simulink model "electrical_model_validation_2015"  (R2015a)
settings: Solver=ode4  StartTime=0.0  StopTime=inf  FixedStep=0.001  RelTol=1e-3
libraries: PoliArd x7
settings Model: CovHtmlReporting=off  ExtModeTrigDuration=2  Creator=User  LastModifiedBy=User
settings OptimizationCC: OptimizeModelRefInitCode=on  LifeSpan=1
settings DebuggingCC: UnderspecifiedInitializationDetection=Classic  MergeDetectMultiDrivingBlocksExec=none
settings HardwareCC: ProdLargestAtomicInteger=Long  ProdLargestAtomicFloat=Double  ProdEndianess=LittleEndian  ProdHWDeviceType=ARM Compatible->ARM Cortex
settings RTWCC: SystemTargetFile=realtime.tlc  GenerateMakefile=off  TemplateMakefile=realtime.tmf  Description=Run on Target Hardware  RTWVerbose=off
settings ERTTargetCC: CombineOutputUpdateFcns=off  ExtModeTransport=3  ExtModeMexFile=ext_serial_win32_comm_rtt  ExtModeMexArgs=0 1 9600  InlinedParameterPlacement=Hierarchical  ERTSrcFileBannerTemplate=realtime_code_template.cgt  ERTHdrFileBannerTemplate=realtime_code_template.cgt  ERTDataSrcFileTemplate=realtime_code_template.cgt  ERTDataHdrFileTemplate=realtime_code_template.cgt  ERTCustomFileTemplate=realtime_file_process.tlc

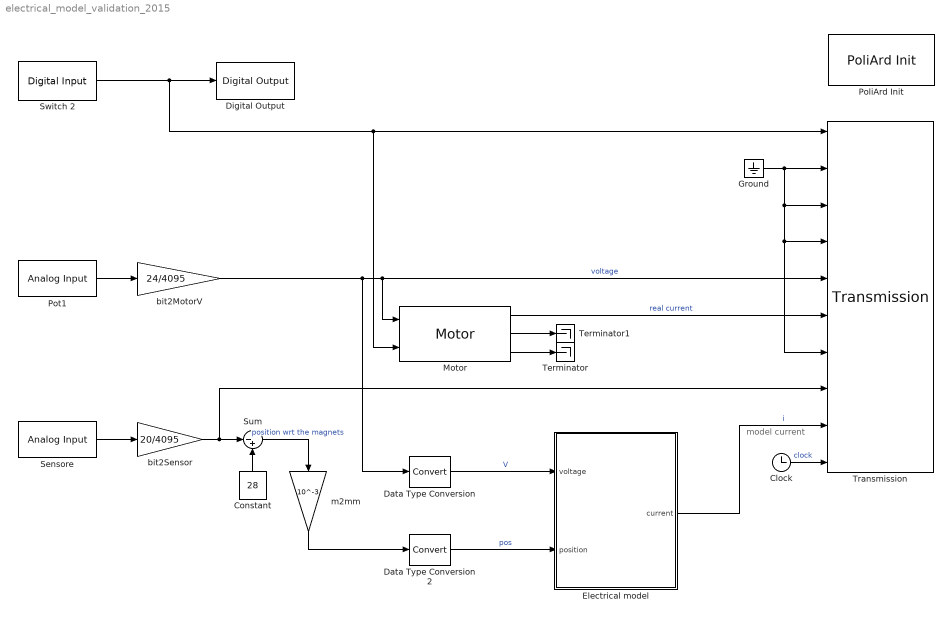
== system electrical_model_validation_2015 ==
  note: model current
  Clock : Clock
  Constant : Constant  Value=28
  Data Type Conversion : DataTypeConversion
  Data Type Conversion2 : DataTypeConversion
  Digital Output : PoliArd/Digital Output  DO_pin=1
  Electrical model : Subsystem
      mask Display: disp('Electrical\nmodel')
  Ground : Ground
  Motor : PoliArd/Motor  MotorID=2  DC_bus_mask=24  dt_mot=-1
  PoliArd Init : PoliArd/PoliArd Init
  Pot1 : PoliArd/Analog Input  AIpin_mask=8  AIsample=-1
  Sensore : PoliArd/Analog Input  AIpin_mask=2  AIsample=-1
  Sum : Sum  Inputs=|-+
  Switch 2 : PoliArd/Digital Input  DI_pin=2  DIsample=-1
  Terminator : Terminator
  Terminator1 : Terminator
  Transmission : PoliArd/Transmission  sample_freq=100  sig_to_send=6
  bit2MotorV : Gain  Gain=24/4095
  bit2Sensor : Gain  Gain=20/4095
  m2mm : Gain  Gain=10^-3
  wires:
  Switch 2/1 -> Motor/2, Transmission/1, Digital Output/1
  Pot1/1 -> bit2MotorV/1
  bit2MotorV/1 -> Data Type Conversion/1, Motor/1, Transmission/5  "voltage"
  Sensore/1 -> bit2Sensor/1
  Ground/1 -> Transmission/7, Transmission/4, Transmission/3, Transmission/2
  Motor/1 -> Transmission/6  "real current"
  Data Type Conversion/1 -> Electrical model/1(voltage)  "V"
  Data Type Conversion2/1 -> Electrical model/2(position)  "pos"
  Electrical model/1(current) -> Transmission/9  "i"
  bit2Sensor/1 -> Transmission/8, Sum/1
  Constant/1 -> Sum/2
  Sum/1 -> m2mm/1  "position wrt the magnets"
  m2mm/1 -> Data Type Conversion2/1
  Clock/1 -> Transmission/10  "clock"
  Motor/3 -> Terminator/1
  Motor/2 -> Terminator1/1

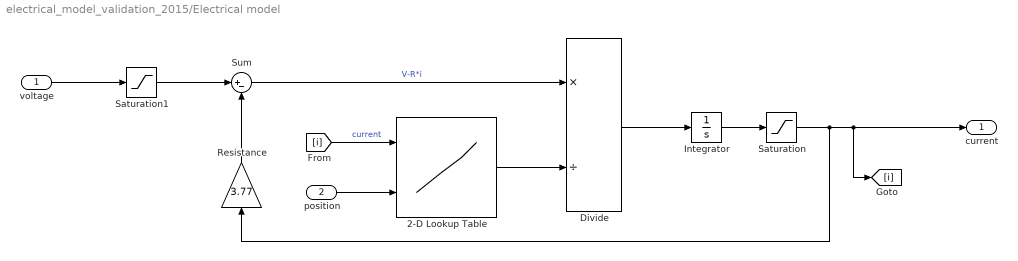
== system electrical_model_validation_2015/Electrical model ==
  voltage : Inport
  position : Inport  Port=2
  2-D Lookup Table : Lookup_n-D  BreakpointsForDimension1="[0.571609272941941\t0.887378665517721\t1.20335132735163\t1.45876147710325\t1.73983455991042\t2.00390586430628\t2.24859052314101\t2.53711534582031\t2.81056000291084\t3.07646645256203\t3.35127777604811\t3.64723023514144\t3.85000000000000]"  BreakpointsForDimension2="[0.00850000000000000\t0.00970000000000000\t0.0105000000000000\t0.0113000000000000\t0.0125000000000000\t0.0135000000000000\t0.0145000000000000\t0.0153000000000000\t0.0165000000000000\t0.0176000000000000\t0.0183000000000000\t0.0198000000000000\t0.0216000000000000\t0.0227000000000000\t0.0236000000000000\t0.0250000000000000]"  Table=|  InternalRulePriority=Speed  RndMeth=Simplest  InputSameDT=on
      | [0.124059778904572	0.115240241777071	0.113604140674407	0.0969706688265998	0.0977224474024037	0.0921484095955819	0.100328887428518	0.0835138746623809	0.0846632562500726	0.101320516519449	0.0850868072661021	0.0849911313704199	0.0770233226672402	0.0728199039666389	0.0857349673426359	0.0658782797079401;
      | 0.149045221919738	0.116659637086155	0.0895561667908866	0.107893626307192	0.125389770928968	0.115549357372873	0.107628431471634	0.0767478700757045	0.113734620814557	0.0487030540411753	0.0854166029154558	0.0852375799265393	0.114494610905458	0.0825536179015005	0.0749113685323473	0.0864552033453527;
      | 0.221473301610230	0.138359268104424	0.127598655408847	0.107655509943492	0.141088050151794	0.102255183896598	0.103076473457404	0.0872435174437226	0.0836166062440565	0.0888634655755324	0.0932839743614151	0.0915177204990435	0.132016146787556	0.0970366780879440	0.0904130771398634	0.108966956576679;
      | 0.223991273176650	0.131524925501924	0.123595637192268	0.117399436946038	0.117485034279105	0.109350617361035	0.103754507171467	0.0861589388580345	0.0857214364348041	0.0917816549943483	0.0890067546609038	0.0816722200620728	0.0814610836052316	0.0767116899255463	0.101900659316609	0.0822633503211632;
      | 0.121687886024072	0.142564456752788	0.125484097705187	0.149105978672514	0.0988303311903818	0.106857219213140	0.0894649045582189	0.0941267712338361	0.142565468524165	0.0818497060473378	0.118301103228728	0.108957534804165	0.106456207125703	0.0760919077107217	0.100144658956964	0.0822619257219681;
      | 0.136138515173081	0.131275746991678	0.174923869014491	0.116373234031288	0.134897498149436	0.147488603603662	0.117217593568497	0.121092621011354	0.0949684484680815	0.120650625212044	0.105528056130615	0.0709218655223650	0.106865162540236	0.112621349170388	0.102672846353554	0.0998828162723997;
      | 0.102540529062246	0.129063716207047	0.128781249629223	0.166531606601018	0.160188607891842	0.143350181522525	0.115424867410468	0.0924580701157953	0.0820347096702044	0.143659809333330	0.0960185227869846	0.0879236610127591	0.119698929732948	0.104624971346943	0.110768236008707	0.103967680724277;
      | 0.0502869330876773	0.0703360930295036	0.121482000910445	0.0868865611541192	0.0998730250371566	0.116253725751726	0.167400667443646	0.161303839871314	0.0985175204299240	0.108488089108738	0.109759635054218	0.0872452567890512	0.125353645131964	0.0875259849372003	0.0849935304722978	0.121626189232489;
      | 0.0210706133138075	0.0515351091202676	0.0426200646343306	0.0565782276211947	0.0745690977819913	0.112020657359165	0.119725047783217	0.0764647313692596	0.142348650861394	0.0639349050075603	0.0904353025903782	0.0861112460202275	0.104664668411399	0.0920235686672933	0.100744620630661	0.106708466661268;
      | 0.0270141671779473	0.0514415556627170	0.0517146134495731	0.0520472356443474	0.0605274494443696	0.0377197714304948	0.0779920314933253	0.0546966093282379	0.106915061624985	0.0869951773796697	0.0883601743545483	0.0742534146214650	0.0717300175437439	0.0897862727514690	0.0997181913290360	0.104066264542440;
      | 0.0233295954754315	0.0449998739143449	0.0266561560962006	0.0155280944859940	0.0317770292575240	0.0319196439820041	0.0527561841503626	0.0297736212828209	0.0370581914149013	0.0386385191066780	0.0587271929401315	0.0453068226188899	0.0773245158334478	0.0738659266965119	0.0647672762562245	0.0535420982543080;
      | 0.0413476484233245	0.0276536768519413	0.0409781731998001	0.0196987497152002	0.0318266325664729	0.0299424263688483	0.0360092728529738	0.0227687678372619	0.0349869001320810	0.0443660538458634	0.0517921958134473	0.0205963949400280	0.0348039807615572	0.0511089243845314	0.0453265105118442	0.0715060082844046;
      | 0.0130190041072452	0.0146415091158683	0.0254138121892464	0.0412159054731432	0.0223960404799849	0.0227241118668500	0.0456462201437789	0.0149368008701184	0.0420919416421131	0.0187588708287234	0.0329663489886674	0.0687911911872538	0.0275417699258336	0.0252373999239683	0.0212106687462740	0.0791031180455345]
  Divide : Product  Inputs=*/
  Integrator : Integrator
  Resistance : Gain  Gain=3.77
  Saturation : Saturate  UpperLimit=3.85  LowerLimit=0
  Saturation1 : Saturate  UpperLimit=15  LowerLimit=0
  Sum : Sum  Inputs=|+-
  current : Outport
  wires:
  Sum/1 -> Divide/1  "V-R*i"
  Integrator/1 -> Saturation/1
  Divide/1 -> Integrator/1
  Resistance/1 -> Sum/2
  Saturation/1 -> current/1, [i], Resistance/1
  voltage/1 -> Saturation1/1
  Saturation1/1 -> Sum/1
  position/1 -> 2-D Lookup Table/2
  2-D Lookup Table/1 -> Divide/2
  [i] -> 2-D Lookup Table/1  "current"
